simulink model "BCI_Arm_Raiser"  (R2023b)
settings: Solver=VariableStepAuto  StartTime=0.0  StopTime=inf  RelTol=1e-3
libraries: hdlsllib x1, vrlib x1
settings Model: Creator=ltcan  LastModifiedBy=ltcan

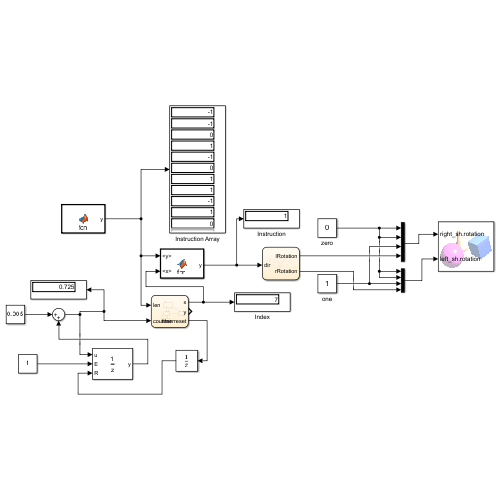
[thumbnail: Simulink's stored preview of the top-level diagram]
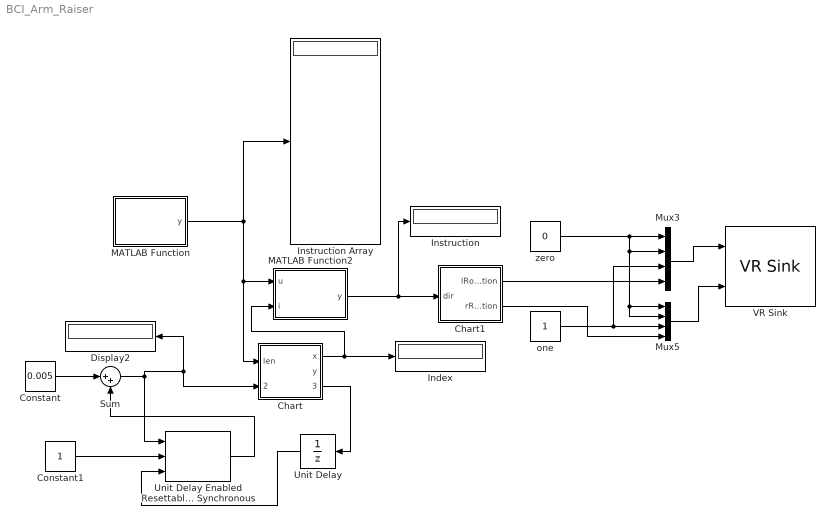
== system BCI_Arm_Raiser ==
  Chart : Stateflow chart  TreatAsAtomicUnit=on
  Chart1 : Stateflow chart  TreatAsAtomicUnit=on
  Constant : Constant  Value=0.005
  Constant1 : Constant
  Display2 : Display
  Index : Display
  Instruction : Display
  Instruction Array : Display
  MATLAB Function : MATLAB Function  TreatAsAtomicUnit=on
  MATLAB Function2 : MATLAB Function  TreatAsAtomicUnit=on
  Mux3 : Mux
  Mux5 : Mux
  Sum : Sum  Inputs=|++
  Unit Delay : UnitDelay  SampleTime=-1  HasFrameUpgradeWarning=on
  Unit Delay Enabled Resettable Synchronous : hdlsllib/Discrete/Unit Delay Enabled Resettable Synchronous  InitialCondition=0.0  SampleTime=-1
  VR Sink : vrlib/VR Sink  InstantiateOnLoad=on  SampleTime=0.1  ViewEnable=on  RemoteChange=off  RemoteView=off  FieldsWritten=right_sh.rotation.4.1.1.double#left_sh.rotation.4.1.1.double  WorldFileName=HW.wrl  AutoView=off  VideoDimensions=[]  AllowVariableSize=off  FigureProperties="{'Position', 'Name', 'Viewpoint', 'CameraBound', 'CameraDirection', 'CameraPosition', 'CameraUpVector', 'ZoomFactor', 'Antialiasing', 'Headlight', 'Lighting', 'NavPanel', 'Sound', 'StatusBar', 'Stereo3D', 'Stereo3DCameraOffset', 'Stereo3DHIT', 'ToolBar', 'Textures', 'Transparency', 'Triad', 'Wireframe', 'NavZones', 'NavMode', 'NavSpeed', 'CaptureFileFormat', 'CaptureFileName', 'Record2DCompressMethod', 'Record2DCompressQuality', 'Record2D', 'Record2DFileName', 'Record2DFPS'; [9.6340000000000009e+02   2.4620000000000005e+02   5.7600000000000000e+02   3.5000000000000000e+02], '', '', 'on', [-2.5276977035525133e-03   0.0000000000000000e+00  -9.9999680536705693e-01], [-8.0718523973111189e-04   1.4438536167144775e+00   9.6806648754176123e+00], [0.0000000000000000e+00   1.0000000000000000e+00   0.0000000000000000e+00], [1.0000000000000000e+00], 'on', 'on', 'on', 'halfbar', 'on', 'on', 'off', [1.0000000149011612e-01], [0.0000000000000000e+00], 'on', 'on', 'on', 'none', 'off', 'off', 'fly', 'normal', 'tif', '%f_anim_%n.tif', 'auto', [7.5000000000000000e+01], 'off', '%f_anim_%n.avi', 'auto'}"
  one : Constant
  zero : Constant  Value=0
  wires:
  one/1 -> Mux3/3, Mux5/3
  zero/1 -> Mux5/2, Mux5/1, Mux3/2, Mux3/1
  Chart1/1(lRotation) -> Mux3/4
  Chart1/2(rRotation) -> Mux5/4
  Sum/1 -> Display2/1, Chart/2(counter), Unit Delay Enabled Resettable Synchronous/1
  Unit Delay Enabled Resettable Synchronous/1 -> Sum/2
  Chart/1(x) -> Index/1, MATLAB Function2/2(i)
  Constant/1 -> Sum/1
  Unit Delay/1 -> Unit Delay Enabled Resettable Synchronous/3
  Constant1/1 -> Unit Delay Enabled Resettable Synchronous/2
  Chart/3(timerreset) -> Unit Delay/1
  MATLAB Function2/1(y) -> Instruction/1, Chart1/1(dir)
  MATLAB Function/1(y) -> Instruction Array/1, Chart/1(len), MATLAB Function2/1(u)
  Mux3/1 -> VR Sink/1
  Mux5/1 -> VR Sink/2

== matlab function BCI_Arm_Raiser/MATLAB Function ==
  data: y output
function y = fcn
% Load commands generated from SVM classifier
x = load('C:/Users/ltcan/Documents/BCI Research/Project Code/Outputs/Filtered data/svm_model.mat', 'commands');
cmds = x.commands;
arr = zeros(1,length(cmds));

for i = 1:length(cmds)
    command = cmds{i};
    if strcmp(command, 'LEFT')
        % Left arm raised
        arr(i) = -1;
    
    elseif strcmp(command, 'RIGHT')
        % Right arm raised
        arr(i) = 1;
    
    else
        % REST — both arms down
        arr(i) = 0;
    end
end
y = arr;

== stateflow chart BCI_Arm_Raiser/Chart ==
  state start
    y = 0;
    x=1;
    timerreset = 0;
  state inc
    y= y + 1;
    timerreset = 1;
  state res
    y=0;
  state set
    x=y;
    timerreset = 0;
  (default) -> start
  start -> inc
  res -> inc
  inc -> res [order 1] : [y > length(len)]
  inc -> set [order 2] : [y <= length(len)]
  set -> inc : [counter > 5]
  data: len input; x output; y output; timerreset output; counter input

== matlab function BCI_Arm_Raiser/MATLAB Function2 ==
  data: u input; i input; y output
function y= fcn(u, i)
y = u(min(i, length(u)));

== stateflow chart BCI_Arm_Raiser/Chart1 ==
  state startState
    lRotation = 0;
    rRotation = 0;
  state centerState
    lRotation = 0;
    rRotation = 0;
  state lRaise
    lRotation = lRotation - 0.01;
    rRotation = 0;
  state rRaise
    lRotation = 0;
    rRotation = rRotation + 0.01;
  state rLower
    lRotation = 0;
    rRotation = rRotation - 0.01;
  state lLower
    lRotation = lRotation + 0.01;
    rRotation = 0;
  state allLower
    lRotation = lRotation + 0.01;
    rRotation = rRotation - 0.01;
  state rRaiseLower
    lRotation = lRotation + 0.01;
    rRotation = rRotation + 0.01;
  state leftRaise
    lRotation = -3;
    rRotation = 0;
  state lRaiseLower
    lRotation = lRotation - 0.01;
    rRotation = rRotation - 0.01;
  state rightRaise
    lRotation = 0;
    rRotation = 3;
  (default) -> startState
  startState -> centerState
  centerState -> rRaise [order 1] : [dir >= 1]
  centerState -> lRaise [order 2] : [dir <= -1]
  lLower -> centerState [order 1] : [dir < 1 && dir > -1 && lRotation >= 0 && rRotation <=0]
  allLower -> centerState [order 1] : [dir < 1 && dir > -1 && lRotation >= 0 && rRotation <= 0]
  rLower -> centerState [order 1] : [dir < 1 && dir > -1 && lRotation >= 0 && rRotation <=0]
  lLower -> lRaise [order 3] : [dir <= -1]
  lRaise -> leftRaise [order 1] : [lRotation <= -3]
  lRaise -> rRaiseLower [order 3] : [dir >= 1]
  lRaiseLower -> lRaise [order 3] : [dir <= -1 && lRotation > -3 && rRotation <= 0]
  lRaise -> lLower [order 2] : [dir < 1 && dir > -1]
  rRaise -> rightRaise [order 1] : [rRotation >= 3]
  rLower -> rRaise [order 3] : [dir >= 1]
  rRaise -> lRaiseLower [order 3] : [dir <= -1]
  rRaiseLower -> rRaise [order 3] : [dir >= 1 && lRotation >= 0 && rRotation < 3]
  rRaise -> rLower [order 2] : [dir < 1 && dir > -1]
  allLower -> rLower [order 2] : [dir < 1 && dir > -1 && lRotation >= 0 && rRotation > 0]
  rLower -> lRaiseLower [order 2] : [dir <= -1]
  rightRaise -> rLower [order 1] : [dir < 1 && dir > -1]
  leftRaise -> lLower [order 1] : [dir > -1 && dir < 1]
  lLower -> rRaiseLower [order 2] : [dir >= 1]
  allLower -> lLower [order 3] : [dir < 1 && dir > -1 && lRotation < 0 && rRotation <= 0]
  allLower -> lRaiseLower [order 5] : [dir <= -1]
  rRaiseLower -> allLower [order 2] : [dir < 1 && dir > -1]
  lRaiseLower -> allLower [order 2] : [dir < 1 && dir > -1]
  allLower -> rRaiseLower [order 4] : [dir >= 1]
  leftRaise -> rRaiseLower [order 2] : [dir >= 1]
  rRaiseLower -> lRaiseLower [order 4] : [dir <= -1 && lRotation > -3 && rRotation > 0]
  lRaiseLower -> rRaiseLower [order 4] : [dir >= 1 && lRotation < 0 && rRotation < 3]
  rRaiseLower -> rightRaise [order 1] : [dir >= 1 && lRotation >= 0 && rRotation >= 3]
  lRaiseLower -> leftRaise [order 1] : [dir <= -1 && lRotation <= -3 && rRotation <= 0]
  rightRaise -> lRaiseLower [order 2] : [dir <= -1]
  data: lRotation output; rRotation output; dir input
